simulink model "gm_sampleModel1840_5_sub"  (R2023a)
settings: Solver=VariableStepAuto  StartTime=0.0  StopTime=10.0  RelTol=1e-3
libraries: hdlsllib x3, simulink x2
settings Model: Creator=user1  LastModifiedBy=user1
settings OptimizationCC: BlockReduction=off  ConditionallyExecuteInputs=off
settings DebuggingCC: InheritedTsInSrcMsg=none

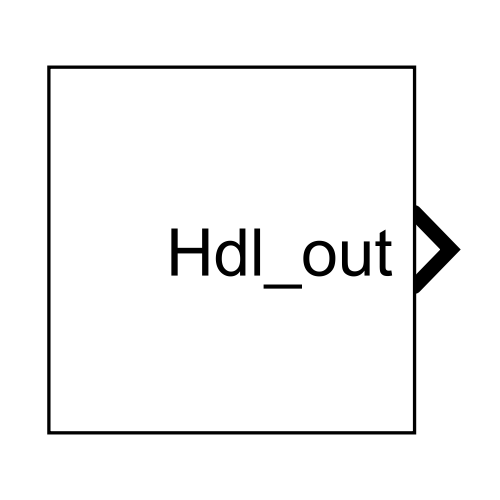
[thumbnail: Simulink's stored preview of the top-level diagram]
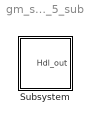
== system gm_sampleModel1840_5_sub ==
  Subsystem : Subsystem

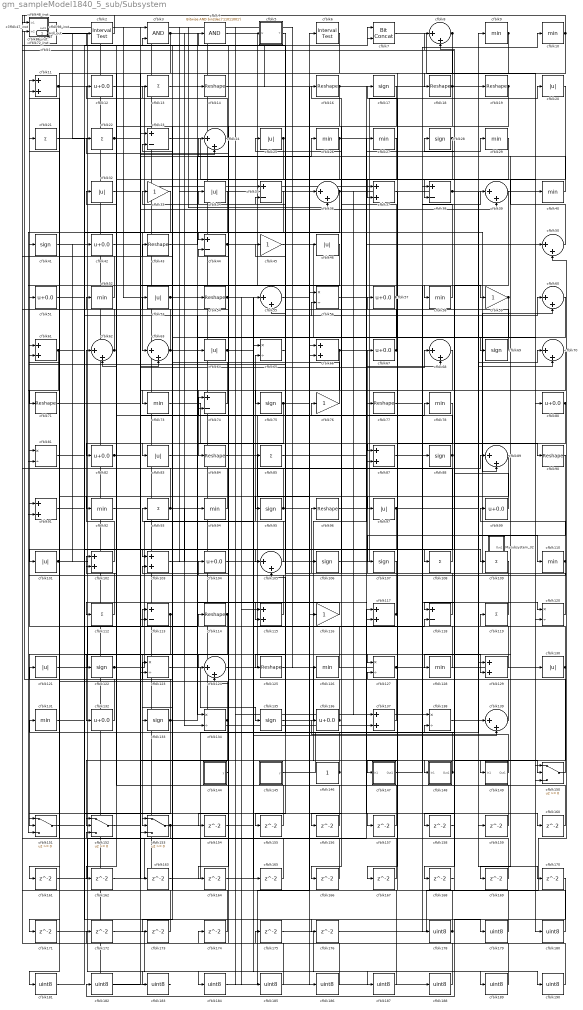
== system gm_sampleModel1840_5_sub/Subsystem ==
  Mysubsystem_32 : Subsystem
  cfblk1 : simulink/Logic and Bit Operations/Bit Clear  iBit=0
      settings: LibrarySourceBlock=|
      | hdlsllib/Logic and Bit
      | Operations/Bit Clear
  cfblk{9..10,26..27,29,40,52,58,73,78,92,94,110,126,128,131} (16 alike) : MinMax  OutDataTypeStr=uint8
  cfblk100_inst : Subsystem
  cfblk{20,25,32,34,46,53,64,83,97,101,121,130} (12 alike) : Abs  OutDataTypeStr=uint8  SaturateOnIntegerOverflow=off
  cfblk{11,37,61,66,87,91,102..103,115,117,129,137} (12 alike) : Sum  OutDataTypeStr=uint8
  cfblk{12,42,51,57,67,80,82,99,104,132,136} (11 alike) : Bias  Bias=0.0  SaturateOnIntegerOverflow=off
  cfblk{8,24,36,39,50,55,60,62..63,68,70,89,105,124,139} (15 alike) : Sum  Inputs=|++  OutDataTypeStr=uint8
  cfblk{17,28,41,69,75,88,95,106..107,122,133,135} (12 alike) : Signum
  cfblk{13,21..22,85,93,108..109,112,119} (9 alike) : Sum  Inputs=+  OutDataTypeStr=uint8
  cfblk111_inst : Subsystem
  cfblk{23,35,38,44,74,113,118} (7 alike) : Sum  Inputs=+-  OutDataTypeStr=uint8
  cfblk{14,16,18..19,43,54,71,77,84,90,96,114,125} (13 alike) : Reshape
  cfblk{33,45,59,76,116} (5 alike) : Gain  OutDataTypeStr=uint8
  cfblk{56,65,81,120,123,127,134,138} (8 alike) : Product  Inputs=*/  OutDataTypeStr=uint8  RndMeth=Zero  SaturateOnIntegerOverflow=on
  cfblk141_inst : Subsystem
  cfblk144 : Subsystem  mask(Counter Free-Running){NumBits=double(16), tsamp=double(-1)}
      mask prompts: NumBits "Simulink:masks:NumberOfBits_MP"; tsamp "Simulink:masks:SampleTime_MP"
      mask help: Simulink:masks:CounterFreeRunning_MD
  cfblk145 : Subsystem  mask(Counter Limited){uplimit=double(7), tsamp=double(-1)}
      mask prompts: uplimit "Simulink:masks:UpperLimit_MP"; tsamp "Simulink:masks:SampleTime_MP"
      mask help: Simulink:masks:CounterLimited_MD
      mask init:
      | nbits = double(8);
      | tsamp = double(-1);
      | uplimit = double(7);
  cfblk146 : Constant  OutDataTypeStr=uint8  SampleTime=-1
  cfblk147 : Subsystem
  cfblk148 : Subsystem
  cfblk149 : Subsystem
  cfblk{150..153} (4 alike) : Switch  OutDataTypeStr=uint8  SaturateOnIntegerOverflow=off  InputSameDT=off
  cfblk{154..176} (23 alike) : Delay  SampleTime=1
  cfblk15_inst : Subsystem
  cfblk{178..190} (13 alike) : DataTypeConversion  OutDataTypeStr=uint8  SaturateOnIntegerOverflow=off  RndMeth=Floor
  cfblk2 : hdlsllib/Logic and Bit Operations/Interval Test  IntervalClosedRight=on  uplimit=0.5  IntervalClosedLeft=on  lowlimit=-0.5  OutDataTypeStr=uint8
  cfblk3 : Logic  AllPortsSameDT=off  OutDataTypeStr=boolean
  cfblk31_inst : Subsystem
  cfblk4 : simulink/Logic and Bit Operations/Bitwise Operator  logicop=AND  UseBitMask=on  BitMask=bin2dec('11011001')  BitMaskRealWorld=Stored Integer
      settings: LibrarySourceBlock=|
      | hdlsllib/Logic and Bit
      | Operations/Bitwise
      | Operator
  cfblk47_inst : Subsystem
  cfblk48_inst : Subsystem
  cfblk5 : Subsystem  mask(Detect Rise Nonnegative){vinit=double(0), InputProcessing=Elements as channels (sample based), OutDataTypeStr=uint8}
      mask prompts: vinit "Simulink:masks:InitialCondition_MP"; InputProcessing "Simulink:masks:InputProcessing_MP"; OutDataTypeStr "Simulink:masks:OutputDataType_MP"
      mask help: Simulink:masks:DetectRiseNonnegative_MD
      mask init:
      | InputProcessing = 'Elements as channels (sample based)';
      | OutDataTypeStr = 'uint8';
      | vinit = double(0);
      mask TypeOptions InputProcessing: Simulink:masks:ColumnsAsChannelsFrameBased | Simulink:masks:ElementsAsChannelsSampleBased
      mask TypeOptions OutDataTypeStr: Simulink:masks:uint8 | Simulink:masks:boolean
      mask Display: fprintf('U >= 0\n&  NOT\nU/z >= 0')
  cfblk6 : hdlsllib/Logic and Bit Operations/Interval Test  IntervalClosedRight=on  uplimit=0.5  IntervalClosedLeft=on  lowlimit=-0.5  OutDataTypeStr=uint8
  cfblk7 : hdlsllib/Logic and Bit Operations/Bit Concat  numInputs=2
  cfblk72_inst : Subsystem
  cfblk86_inst : Subsystem
  cfblk98_inst : Subsystem
  Hdl_out : Outport  OutDataTypeStr=uint8  SampleTime=1
  wires:
  Mysubsystem_32/1(Out1) -> cfblk128/1
  cfblk1/1 -> cfblk184/1
  cfblk10/1 -> cfblk98_inst/1(in1), cfblk18/1
  cfblk100_inst/1(out1) -> cfblk36/1, cfblk19/1
  cfblk101/1 -> cfblk42/1, cfblk129/2
  cfblk102/1 -> cfblk62/1
  cfblk103/1 -> cfblk94/1
  cfblk104/1 -> cfblk76/1
  cfblk105/1 -> cfblk65/2
  cfblk106/1 -> cfblk20/1
  cfblk107/1 -> cfblk96/1
  cfblk108/1 -> cfblk48_inst/1(in1)
  cfblk109/1 -> cfblk60/2
  cfblk11/1 -> cfblk63/1, cfblk139/1
  cfblk110/1 -> cfblk99/1, cfblk104/1
  cfblk111_inst/1(out1) -> cfblk165/1
  cfblk112/1 -> cfblk102/1
  cfblk113/1 -> cfblk43/1, cfblk132/1
  cfblk114/1 -> cfblk153/2, cfblk151/2
  cfblk115/1 -> cfblk11/1
  cfblk116/1 -> cfblk112/1
  cfblk117/1 -> cfblk16/1, cfblk93/1
  cfblk118/1 -> cfblk61/1
  cfblk119/1 -> cfblk67/1
  cfblk12/1 -> cfblk89/2
  cfblk120/1 -> cfblk34/1
  cfblk121/1 -> cfblk64/1
  cfblk122/1 -> cfblk63/2, cfblk65/1
  cfblk123/1 -> cfblk135/1
  cfblk124/1 -> cfblk89/1
  cfblk125/1 -> cfblk148/1(In1)
  cfblk126/1 -> cfblk52/1
  cfblk127/1 -> cfblk57/1, cfblk17/1, cfblk10/1
  cfblk128/1 -> cfblk13/1
  cfblk129/1 -> cfblk91/1
  cfblk13/1 -> cfblk134/1
  cfblk130/1 -> cfblk168/1, cfblk119/1
  cfblk131/1 -> cfblk153/1
  cfblk132/1 -> cfblk121/1
  cfblk133/1 -> cfblk98_inst/2(in2), cfblk171/1, cfblk78/1
  cfblk134/1 -> cfblk152/2, cfblk81/1
  cfblk135/1 -> cfblk27/1
  cfblk136/1 -> cfblk51/1, cfblk15_inst/2(in2)
  cfblk137/1 -> cfblk103/2
  cfblk138/1 -> cfblk70/2
  cfblk139/1 -> cfblk33/1
  cfblk14/1 -> cfblk66/2
  cfblk141_inst/1(out1) -> cfblk188/1
  cfblk144/1(y) -> cfblk114/1
  cfblk145/1(y) -> cfblk9/1
  cfblk146/1 -> cfblk11/2, cfblk131/1
  cfblk147/1(Out1) -> cfblk39/1
  cfblk148/1(Out1) -> cfblk53/1, cfblk105/2
  cfblk149/1(Out1) -> cfblk136/1
  cfblk15_inst/1(out1) -> cfblk130/1, cfblk106/1
  cfblk150/1 -> cfblk22/1
  cfblk151/1 -> cfblk157/1
  cfblk152/1 -> cfblk24/2
  cfblk153/1 -> cfblk152/3, cfblk129/1
  cfblk154/1 -> cfblk55/1
  cfblk155/1 -> cfblk102/2
  cfblk156/1 -> cfblk62/2
  cfblk157/1 -> cfblk44/2
  cfblk158/1 -> cfblk8/2
  cfblk159/1 -> cfblk23/2
  cfblk16/1 -> cfblk150/2, cfblk115/2
  cfblk160/1 -> cfblk3/2
  cfblk161/1 -> cfblk117/1
  cfblk162/1 -> cfblk66/1
  cfblk163/1 -> cfblk70/1
  cfblk164/1 -> cfblk118/2
  cfblk165/1 -> cfblk61/2
  cfblk166/1 -> cfblk100_inst/2(in2)
  cfblk167/1 -> cfblk113/1
  cfblk168/1 -> cfblk138/2
  cfblk169/1 -> cfblk15_inst/1(in1)
  cfblk17/1 -> cfblk162/1
  cfblk170/1 -> cfblk182/1
  cfblk171/1 -> cfblk183/1
  cfblk172/1 -> cfblk187/1
  cfblk173/1 -> cfblk86_inst/2(in2)
  cfblk174/1 -> cfblk123/1
  cfblk175/1 -> cfblk189/1
  cfblk176/1 -> cfblk50/2
  cfblk178/1 -> cfblk72_inst/2(in2), cfblk127/2
  cfblk179/1 -> cfblk77/1
  cfblk18/1 -> cfblk125/1, cfblk111_inst/2(in2), cfblk166/1
  cfblk180/1 -> cfblk28/1
  cfblk181/1 -> cfblk7/1
  cfblk182/1 -> cfblk7/2
  cfblk183/1 -> cfblk1/1
  cfblk184/1 -> cfblk6/1
  cfblk185/1 -> cfblk4/1
  cfblk186/1 -> cfblk174/1
  cfblk187/1 -> cfblk31_inst/1(in1)
  cfblk188/1 -> cfblk172/1
  cfblk189/1 -> cfblk48_inst/2(in2)
  cfblk19/1 -> cfblk133/1, cfblk124/1
  cfblk190/1 -> cfblk175/1
  cfblk2/1 -> cfblk72_inst/1(in1)
  cfblk20/1 -> cfblk169/1
  cfblk21/1 -> cfblk109/1
  cfblk22/1 -> Hdl_out/1, cfblk58/1
  cfblk23/1 -> cfblk80/1
  cfblk24/1 -> cfblk12/1
  cfblk25/1 -> cfblk122/1, cfblk92/1
  cfblk26/1 -> cfblk83/1, cfblk68/2
  cfblk27/1 -> cfblk75/1
  cfblk28/1 -> cfblk38/2, cfblk123/2
  cfblk29/1 -> cfblk95/1
  cfblk3/1 -> cfblk113/2, cfblk105/1, cfblk134/2
  cfblk31_inst/1(out1) -> cfblk141_inst/2(in2), cfblk141_inst/1(in1), cfblk137/2, cfblk138/1, cfblk40/1
  cfblk32/1 -> cfblk59/1
  cfblk33/1 -> cfblk181/1
  cfblk34/1 -> cfblk73/1
  cfblk35/1 -> cfblk161/1
  cfblk36/1 -> cfblk91/2, cfblk137/1
  cfblk37/1 -> cfblk167/1
  cfblk38/1 -> cfblk159/1, cfblk110/1
  cfblk39/1 -> cfblk158/1
  cfblk4/1 -> cfblk186/1
  cfblk40/1 -> cfblk24/1
  cfblk41/1 -> cfblk44/1
  cfblk42/1 -> cfblk149/1(In1)
  cfblk43/1 -> cfblk26/1
  cfblk44/1 -> cfblk88/1, cfblk154/1
  cfblk45/1 -> cfblk120/2
  cfblk46/1 -> cfblk81/2
  cfblk47_inst/1(out1) -> cfblk35/1
  cfblk48_inst/1(out1) -> cfblk54/1, cfblk36/2
  cfblk5/1(Y) -> cfblk155/1
  cfblk50/1 -> cfblk23/1
  cfblk51/1 -> cfblk179/1
  cfblk52/1 -> cfblk100_inst/1(in1)
  cfblk53/1 -> cfblk87/1, cfblk69/1
  cfblk54/1 -> cfblk190/1, cfblk185/1
  cfblk55/1 -> cfblk116/1
  cfblk56/1 -> cfblk160/1
  cfblk57/1 -> cfblk25/1, cfblk164/1
  cfblk58/1 -> cfblk38/1
  cfblk59/1 -> cfblk103/1, cfblk156/1
  cfblk6/1 -> cfblk55/2
  cfblk60/1 -> cfblk87/2
  cfblk61/1 -> cfblk3/1, cfblk151/3
  cfblk62/1 -> cfblk86_inst/1(in1), cfblk21/1
  cfblk63/1 -> cfblk47_inst/1(in1), cfblk56/2
  cfblk64/1 -> cfblk139/2, cfblk115/1, cfblk176/1
  cfblk65/1 -> cfblk45/1
  cfblk66/1 -> cfblk153/3, cfblk29/1
  cfblk67/1 -> cfblk35/2, cfblk147/1(In1)
  cfblk68/1 -> cfblk173/1
  cfblk69/1 -> cfblk111_inst/1(in1)
  cfblk7/1 -> cfblk180/1
  cfblk70/1 -> cfblk84/1
  cfblk71/1 -> cfblk39/2
  cfblk72_inst/1(out1) -> cfblk5/1(U)
  cfblk73/1 -> cfblk150/1
  cfblk74/1 -> cfblk31_inst/2(in2)
  cfblk75/1 -> cfblk90/1, cfblk82/1
  cfblk76/1 -> cfblk41/1
  cfblk77/1 -> cfblk178/1
  cfblk78/1 -> cfblk97/1
  cfblk8/1 -> cfblk71/1, cfblk152/1
  cfblk80/1 -> cfblk150/3, cfblk118/1
  cfblk81/1 -> cfblk60/1
  cfblk82/1 -> cfblk74/1, cfblk68/1
  cfblk83/1 -> cfblk117/2
  cfblk84/1 -> cfblk126/1
  cfblk85/1 -> cfblk50/1
  cfblk86_inst/1(out1) -> cfblk14/1
  cfblk87/1 -> cfblk120/1
  cfblk88/1 -> cfblk32/1, cfblk124/2
  cfblk89/1 -> cfblk151/1
  cfblk9/1 -> cfblk74/2, cfblk37/2
  cfblk90/1 -> cfblk107/1
  cfblk91/1 -> cfblk127/1
  cfblk92/1 -> cfblk163/1
  cfblk93/1 -> cfblk47_inst/2(in2), cfblk56/1
  cfblk94/1 -> cfblk2/1
  cfblk95/1 -> cfblk46/1, cfblk85/1
  cfblk96/1 -> cfblk108/1
  cfblk97/1 -> cfblk101/1, cfblk170/1
  cfblk98_inst/1(out1) -> cfblk37/1
  cfblk99/1 -> cfblk8/1

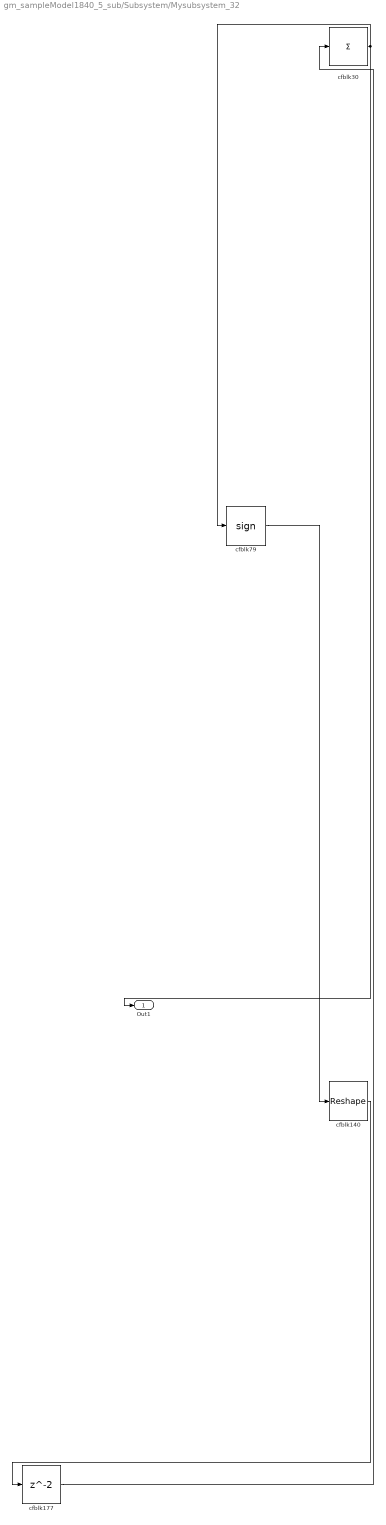
== system gm_sampleModel1840_5_sub/Subsystem/Mysubsystem_32 ==
  cfblk140 : Reshape
  cfblk177 : Delay  SampleTime=1
  cfblk30 : Sum  Inputs=+
  cfblk79 : Signum
  Out1 : Outport  SampleTime=1
  wires:
  cfblk140/1 -> cfblk177/1
  cfblk177/1 -> cfblk30/1
  cfblk30/1 -> cfblk79/1, Out1/1
  cfblk79/1 -> cfblk140/1

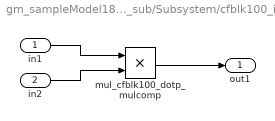
== system gm_sampleModel1840_5_sub/Subsystem/cfblk100_inst ==
  in1 : Inport  OutDataTypeStr=uint8  SampleTime=1
  in2 : Inport  Port=2  OutDataTypeStr=uint8  SampleTime=1
  mul_cfblk100_dotp_mulcomp : Product  Inputs=**  OutDataTypeStr=uint8  SampleTime=1
  out1 : Outport  OutDataTypeStr=uint8  SampleTime=1
  wires:
  in1/1 -> mul_cfblk100_dotp_mulcomp/1
  in2/1 -> mul_cfblk100_dotp_mulcomp/2
  mul_cfblk100_dotp_mulcomp/1 -> out1/1

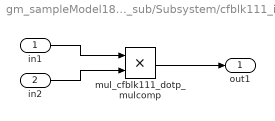
== system gm_sampleModel1840_5_sub/Subsystem/cfblk111_inst ==
  in1 : Inport  OutDataTypeStr=uint8  SampleTime=1
  in2 : Inport  Port=2  OutDataTypeStr=uint8  SampleTime=1
  mul_cfblk111_dotp_mulcomp : Product  Inputs=**  OutDataTypeStr=uint8  SampleTime=1
  out1 : Outport  OutDataTypeStr=uint8  SampleTime=1
  wires:
  in1/1 -> mul_cfblk111_dotp_mulcomp/1
  in2/1 -> mul_cfblk111_dotp_mulcomp/2
  mul_cfblk111_dotp_mulcomp/1 -> out1/1

== system gm_sampleModel1840_5_sub/Subsystem/cfblk141_inst ==
  in1 : Inport  OutDataTypeStr=uint8  SampleTime=1
  in2 : Inport  Port=2  OutDataTypeStr=uint8  SampleTime=1
  mul_cfblk141_dotp_mulcomp : Product  Inputs=**  OutDataTypeStr=uint8  SampleTime=1
  out1 : Outport  OutDataTypeStr=uint8  SampleTime=1
  wires:
  in1/1 -> mul_cfblk141_dotp_mulcomp/1
  in2/1 -> mul_cfblk141_dotp_mulcomp/2
  mul_cfblk141_dotp_mulcomp/1 -> out1/1

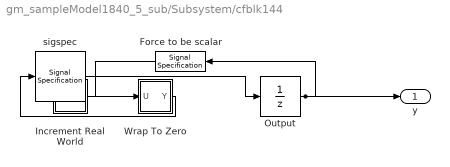
== system gm_sampleModel1840_5_sub/Subsystem/cfblk144 ==
  Force to be scalar : SignalSpecification  DisableCoverage=on  Dimensions=1
  Increment Real World : Subsystem  mask(Real World Value Increment){}
      mask help: Simulink:masks:RealWorldValueIncrement_MD
      mask Display: disp('V++')
  Output : UnitDelay  InitialCondition=0.0  SampleTime=tsamp  HasFrameUpgradeWarning=on
  Wrap To Zero : Subsystem  mask(Wrap To Zero){Threshold=double(65535)}
      mask prompts: Threshold "Simulink:masks:Threshold_MP"
      mask help: Simulink:masks:WrapToZero_MD
  sigspec : SignalSpecification  OutDataTypeStr=uint16  Dimensions=1
  y : Outport  SampleTime=1
  wires:
  Force to be scalar/1 -> Increment Real World/1(u)
  Increment Real World/1(y) -> Wrap To Zero/1(U)
  Output/1 -> Force to be scalar/1, y/1
  Wrap To Zero/1(Y) -> sigspec/1
  sigspec/1 -> Output/1

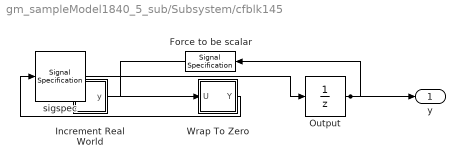
== system gm_sampleModel1840_5_sub/Subsystem/cfblk145 ==
  Force to be scalar : SignalSpecification  DisableCoverage=on  Dimensions=1
  Increment Real World : Subsystem  mask(Real World Value Increment){}
      mask help: Simulink:masks:RealWorldValueIncrement_MD
      mask Display: disp('V++')
  Output : UnitDelay  InitialCondition=0.0  SampleTime=tsamp  HasFrameUpgradeWarning=on
  Wrap To Zero : Subsystem  mask(Wrap To Zero){Threshold=double(7)}
      mask prompts: Threshold "Simulink:masks:Threshold_MP"
      mask help: Simulink:masks:WrapToZero_MD
  sigspec : SignalSpecification  OutDataTypeStr=uint8  Dimensions=1
  y : Outport  SampleTime=1
  wires:
  Force to be scalar/1 -> Increment Real World/1(u)
  Increment Real World/1(y) -> Wrap To Zero/1(U)
  Output/1 -> Force to be scalar/1, y/1
  Wrap To Zero/1(Y) -> sigspec/1
  sigspec/1 -> Output/1

== system gm_sampleModel1840_5_sub/Subsystem/cfblk147 ==
  In1 : Inport  OutDataTypeStr=uint8  PortDimensions=1  SampleTime=1
  Out1 : Outport  SampleTime=1
  wires:
  In1/1 -> Out1/1

== system gm_sampleModel1840_5_sub/Subsystem/cfblk148 ==
  In1 : Inport  OutDataTypeStr=uint8  PortDimensions=1  SampleTime=1
  Out1 : Outport  SampleTime=1
  wires:
  In1/1 -> Out1/1

== system gm_sampleModel1840_5_sub/Subsystem/cfblk149 ==
  In1 : Inport  OutDataTypeStr=uint8  PortDimensions=1  SampleTime=1
  Out1 : Outport  SampleTime=1
  wires:
  In1/1 -> Out1/1

== system gm_sampleModel1840_5_sub/Subsystem/cfblk15_inst ==
  in1 : Inport  OutDataTypeStr=uint8  SampleTime=1
  in2 : Inport  Port=2  OutDataTypeStr=uint8  SampleTime=1
  mul_cfblk15_dotp_mulcomp : Product  Inputs=**  OutDataTypeStr=uint8  SampleTime=1
  out1 : Outport  OutDataTypeStr=uint8  SampleTime=1
  wires:
  in1/1 -> mul_cfblk15_dotp_mulcomp/1
  in2/1 -> mul_cfblk15_dotp_mulcomp/2
  mul_cfblk15_dotp_mulcomp/1 -> out1/1

== system gm_sampleModel1840_5_sub/Subsystem/cfblk31_inst ==
  in1 : Inport  OutDataTypeStr=uint8  SampleTime=1
  in2 : Inport  Port=2  OutDataTypeStr=uint8  SampleTime=1
  mul_cfblk31_dotp_mulcomp : Product  Inputs=**  OutDataTypeStr=uint8  SampleTime=1
  out1 : Outport  OutDataTypeStr=uint8  SampleTime=1
  wires:
  in1/1 -> mul_cfblk31_dotp_mulcomp/1
  in2/1 -> mul_cfblk31_dotp_mulcomp/2
  mul_cfblk31_dotp_mulcomp/1 -> out1/1

== system gm_sampleModel1840_5_sub/Subsystem/cfblk47_inst ==
  in1 : Inport  OutDataTypeStr=uint8  SampleTime=1
  in2 : Inport  Port=2  OutDataTypeStr=uint8  SampleTime=1
  mul_cfblk47_dotp_mulcomp : Product  Inputs=**  OutDataTypeStr=uint8  SampleTime=1
  out1 : Outport  OutDataTypeStr=uint8  SampleTime=1
  wires:
  in1/1 -> mul_cfblk47_dotp_mulcomp/1
  in2/1 -> mul_cfblk47_dotp_mulcomp/2
  mul_cfblk47_dotp_mulcomp/1 -> out1/1

== system gm_sampleModel1840_5_sub/Subsystem/cfblk48_inst ==
  in1 : Inport  OutDataTypeStr=uint8  SampleTime=1
  in2 : Inport  Port=2  OutDataTypeStr=uint8  SampleTime=1
  mul_cfblk48_dotp_mulcomp : Product  Inputs=**  OutDataTypeStr=uint8  SampleTime=1
  out1 : Outport  OutDataTypeStr=uint8  SampleTime=1
  wires:
  in1/1 -> mul_cfblk48_dotp_mulcomp/1
  in2/1 -> mul_cfblk48_dotp_mulcomp/2
  mul_cfblk48_dotp_mulcomp/1 -> out1/1

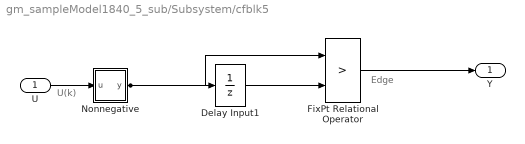
== system gm_sampleModel1840_5_sub/Subsystem/cfblk5 ==
  note: U(k)
  note: Edge
  U : Inport  OutDataTypeStr=uint8  SampleTime=1
  Delay Input1 : UnitDelay  Description=Store in Global RAM  DisableCoverage=on  InitialCondition=vinit  SampleTime=-1  HasFrameUpgradeWarning=on
  FixPt Relational Operator : RelationalOperator  Operator=>  OutDataTypeStr=fixdt(0, 8)  ZeroCross=off  InputSameDT=off
  Nonnegative : Subsystem  mask(Compare To Zero){relop=>=, OutDataTypeStr=boolean, ZeroCross=off}
      mask prompts: relop "Simulink:masks:Operator_MP"; OutDataTypeStr "Simulink:masks:OutputDataType_MP"; ZeroCross "Simulink:masks:EnableZerocrossingDetection_MP"
      mask help: Simulink:masks:CompareToZero_MD
      mask init:
      | OutDataTypeStr = 'boolean';
      | ZeroCross = 'off';
      | blkName = 'sampleModel1840_5_sub/Subsystem/cfblk5/Nonnegative';
      | relop = '>=';
      | setValue = 'boolean';
      mask TypeOptions relop: == | ~= | < | <= | >= | >
      mask TypeOptions OutDataTypeStr: Simulink:masks:uint8 | Simulink:masks:boolean
      mask Callback ZeroCross: sl('zeroCrossEnable', gcbh);
      mask Display: disp([relop,' 0'])
  Y : Outport  SampleTime=1
  wires:
  U/1 -> Nonnegative/1(u)
  Delay Input1/1 -> FixPt Relational Operator/2
  FixPt Relational Operator/1 -> Y/1
  Nonnegative/1(y) -> FixPt Relational Operator/1, Delay Input1/1

== system gm_sampleModel1840_5_sub/Subsystem/cfblk72_inst ==
  in1 : Inport  OutDataTypeStr=uint8  SampleTime=1
  in2 : Inport  Port=2  OutDataTypeStr=uint8  SampleTime=1
  mul_cfblk72_dotp_mulcomp : Product  Inputs=**  OutDataTypeStr=uint8  SampleTime=1
  out1 : Outport  OutDataTypeStr=uint8  SampleTime=1
  wires:
  in1/1 -> mul_cfblk72_dotp_mulcomp/1
  in2/1 -> mul_cfblk72_dotp_mulcomp/2
  mul_cfblk72_dotp_mulcomp/1 -> out1/1

== system gm_sampleModel1840_5_sub/Subsystem/cfblk86_inst ==
  in1 : Inport  OutDataTypeStr=uint8  SampleTime=1
  in2 : Inport  Port=2  OutDataTypeStr=uint8  SampleTime=1
  mul_cfblk86_dotp_mulcomp : Product  Inputs=**  OutDataTypeStr=uint8  SampleTime=1
  out1 : Outport  OutDataTypeStr=uint8  SampleTime=1
  wires:
  in1/1 -> mul_cfblk86_dotp_mulcomp/1
  in2/1 -> mul_cfblk86_dotp_mulcomp/2
  mul_cfblk86_dotp_mulcomp/1 -> out1/1

== system gm_sampleModel1840_5_sub/Subsystem/cfblk98_inst ==
  in1 : Inport  OutDataTypeStr=uint8  SampleTime=1
  in2 : Inport  Port=2  OutDataTypeStr=uint8  SampleTime=1
  mul_cfblk98_dotp_mulcomp : Product  Inputs=**  OutDataTypeStr=uint8  SampleTime=1
  out1 : Outport  OutDataTypeStr=uint8  SampleTime=1
  wires:
  in1/1 -> mul_cfblk98_dotp_mulcomp/1
  in2/1 -> mul_cfblk98_dotp_mulcomp/2
  mul_cfblk98_dotp_mulcomp/1 -> out1/1

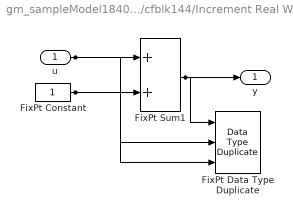
== system gm_sampleModel1840_5_sub/Subsystem/cfblk144/Increment Real World ==
  u : Inport  OutDataTypeStr=uint16  SampleTime=1
  FixPt Constant : Constant  DisableCoverage=on  OutDataTypeStr=Inherit: Inherit via back propagation  SampleTime=-1
  FixPt Data Type Duplicate : DataTypeDuplicate  DisableCoverage=on  NumInputPorts=3
  FixPt Sum1 : Sum  InputSameDT=on  OutDataTypeStr=Inherit: Inherit via back propagation  LockScale=on
  y : Outport  SampleTime=1
  wires:
  u/1 -> FixPt Sum1/1, FixPt Data Type Duplicate/2
  FixPt Constant/1 -> FixPt Sum1/2, FixPt Data Type Duplicate/3
  FixPt Sum1/1 -> FixPt Data Type Duplicate/1, y/1

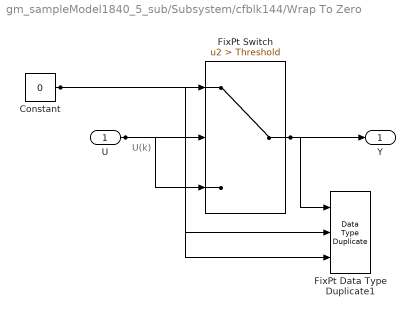
== system gm_sampleModel1840_5_sub/Subsystem/cfblk144/Wrap To Zero ==
  note: U(k)
  U : Inport  OutDataTypeStr=uint16  SampleTime=1
  Constant : Constant  DisableCoverage=on  Value=0  OutDataTypeStr=Inherit: Inherit via back propagation  SampleTime=-1
  FixPt Data Type Duplicate1 : DataTypeDuplicate  DisableCoverage=on  NumInputPorts=3
  FixPt Switch : Switch  Criteria=u2 > Threshold  Threshold=Threshold  OutDataTypeStr=Inherit: Inherit via back propagation  ZeroCross=off  SaturateOnIntegerOverflow=off  InputSameDT=off
  Y : Outport  SampleTime=1
  wires:
  U/1 -> FixPt Switch/3, FixPt Switch/2, FixPt Data Type Duplicate1/2
  Constant/1 -> FixPt Switch/1, FixPt Data Type Duplicate1/3
  FixPt Switch/1 -> FixPt Data Type Duplicate1/1, Y/1

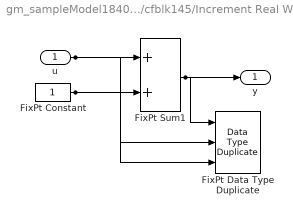
== system gm_sampleModel1840_5_sub/Subsystem/cfblk145/Increment Real World ==
  u : Inport  OutDataTypeStr=uint8  SampleTime=1
  FixPt Constant : Constant  DisableCoverage=on  OutDataTypeStr=Inherit: Inherit via back propagation  SampleTime=-1
  FixPt Data Type Duplicate : DataTypeDuplicate  DisableCoverage=on  NumInputPorts=3
  FixPt Sum1 : Sum  InputSameDT=on  OutDataTypeStr=Inherit: Inherit via back propagation  LockScale=on
  y : Outport  SampleTime=1
  wires:
  u/1 -> FixPt Sum1/1, FixPt Data Type Duplicate/2
  FixPt Constant/1 -> FixPt Sum1/2, FixPt Data Type Duplicate/3
  FixPt Sum1/1 -> FixPt Data Type Duplicate/1, y/1

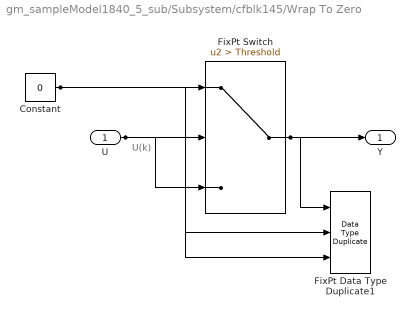
== system gm_sampleModel1840_5_sub/Subsystem/cfblk145/Wrap To Zero ==
  note: U(k)
  U : Inport  OutDataTypeStr=uint8  SampleTime=1
  Constant : Constant  DisableCoverage=on  Value=0  OutDataTypeStr=Inherit: Inherit via back propagation  SampleTime=-1
  FixPt Data Type Duplicate1 : DataTypeDuplicate  DisableCoverage=on  NumInputPorts=3
  FixPt Switch : Switch  Criteria=u2 > Threshold  Threshold=Threshold  OutDataTypeStr=Inherit: Inherit via back propagation  ZeroCross=off  SaturateOnIntegerOverflow=off  InputSameDT=off
  Y : Outport  SampleTime=1
  wires:
  U/1 -> FixPt Switch/3, FixPt Switch/2, FixPt Data Type Duplicate1/2
  Constant/1 -> FixPt Switch/1, FixPt Data Type Duplicate1/3
  FixPt Switch/1 -> FixPt Data Type Duplicate1/1, Y/1

== system gm_sampleModel1840_5_sub/Subsystem/cfblk5/Nonnegative ==
  u : Inport  OutDataTypeStr=uint8  SampleTime=1
  Compare : RelationalOperator  OutDataTypeStr=boolean  ZeroCross=off
  Constant : Constant  DisableCoverage=on  Value=0  OutDataTypeStr=Inherit: Inherit via back propagation  SampleTime=-1  PreserveConstantTs=on
  y : Outport  SampleTime=1
  wires:
  u/1 -> Compare/1
  Compare/1 -> y/1
  Constant/1 -> Compare/2
